simulink model "FLC"  (R2018a)
settings: Solver=VariableStepAuto  StartTime=0.0  StopTime=10  RelTol=1e-3
libraries: fuzblock x1
settings Model: Creator=杨向文  LastModifiedBy=杨向文
settings SolverCC: ZeroCrossAlgorithm=Adaptive

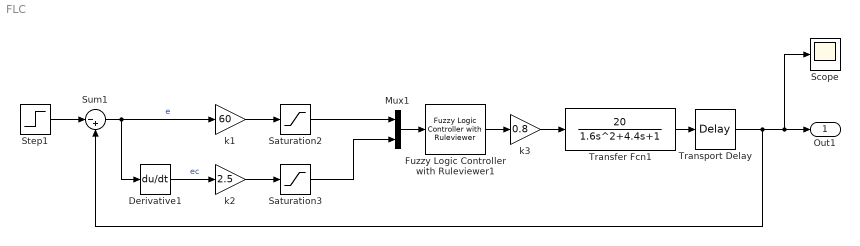
== system FLC ==
  Derivative1 : Derivative
  Fuzzy Logic Controller with Ruleviewer1 : fuzblock/Fuzzy Logic  Controller  with Ruleviewer  fismatrix=flc  Ts=2
  Mux1 : Mux  Inputs=2
  Saturation2 : Saturate  UpperLimit=1  LowerLimit=-1
  Saturation3 : Saturate  UpperLimit=1  LowerLimit=-1
  Scope : Scope
  Step1 : Step  Time=0  SampleTime=0
  Sum1 : Sum  Inputs=|-+
  Transfer Fcn1 : TransferFcn  Numerator=[20]  Denominator=[1.6 4.4 1]
  Transport Delay : TransportDelay  DelayTime=0.02
  k1 : Gain  Gain=60
  k2 : Gain  Gain=2.5
  k3 : Gain  Gain=0.8
  Out1 : Outport
  wires:
  k3/1 -> Transfer Fcn1/1
  Sum1/1 -> Derivative1/1, k1/1  "e"
  Mux1/1 -> Fuzzy Logic Controller with Ruleviewer1/1
  Saturation3/1 -> Mux1/2
  Saturation2/1 -> Mux1/1
  Fuzzy Logic Controller with Ruleviewer1/1 -> k3/1
  Step1/1 -> Sum1/1
  Derivative1/1 -> k2/1  "ec"
  k1/1 -> Saturation2/1
  k2/1 -> Saturation3/1
  Transfer Fcn1/1 -> Transport Delay/1
  Transport Delay/1 -> Scope/1, Out1/1, Sum1/2
